simulink model "model_sim_fuzzy"  (R2023b)
settings: Solver=FixedStepAuto  StartTime=0.0  StopTime=tsim  FixedStep=T  RelTol=1e-3
values from neighbouring files (symbols this model uses):
  GIE = Ki(1) * GE(1)    [gains.m]
  GU = Kp(1) / GE(1)    [gains.m]
undefined symbols (not defined in the file or in its folder): GCE, GE, T
libraries: fuzblock x2
settings Model: Creator=usuario  LastModifiedBy=usuario
settings DataIOCC: ReturnWorkspaceOutputs=off  TimeSaveName=t

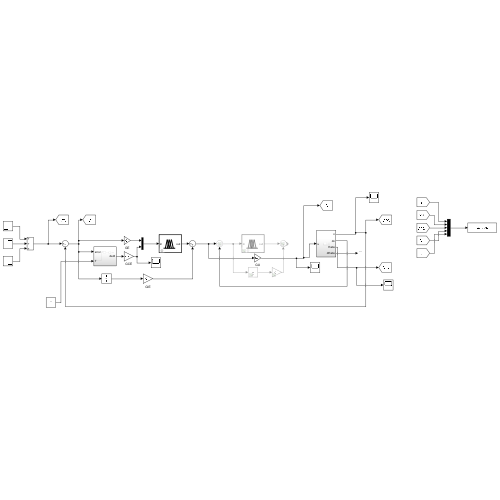
[thumbnail: Simulink's stored preview of the top-level diagram]
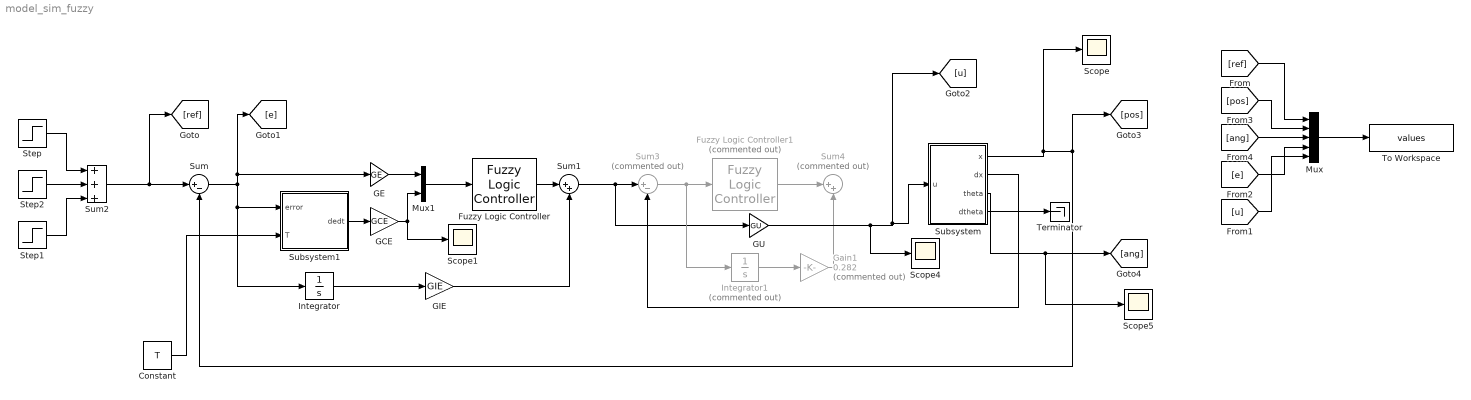
== system model_sim_fuzzy ==
  Constant : Constant  Value=T
  Fuzzy Logic Controller : fuzblock/Fuzzy Logic  Controller  FIS='PID.fis'  OutputSampleNumber=101  DataType=double  FuzzifiedInputs=off  RuleFiringStrengths=off  RuleOutputs=off  AggregatedOutputs=off  SimulateUsing=Interpreted execution  OutOfRangeInputValueMessage=warning  NoRuleFiredMessage=warning  EmptyOutputFuzzySetMessage=warning
  Fuzzy Logic Controller1 : fuzblock/Fuzzy Logic  Controller  Commented=on  FIS='PI.fis'  OutputSampleNumber=101  DataType=double  FuzzifiedInputs=off  RuleFiringStrengths=off  RuleOutputs=off  AggregatedOutputs=off  SimulateUsing=Interpreted execution  OutOfRangeInputValueMessage=warning  NoRuleFiredMessage=warning  EmptyOutputFuzzySetMessage=warning
  GCE : Gain  Gain=GCE
  GE : Gain  Gain=GE
  GIE : Gain  Gain=GIE
  GU : Gain  Gain=GU
  Gain1 : Gain  Commented=on  Gain=0.282
  Integrator : Integrator
  Integrator1 : Integrator  Commented=on
  Mux : Mux  Inputs=5
  Mux1 : Mux  Inputs=2
  Scope{,1,4..5} (4 alike) : Scope
  Step : Step  Time=0  After=0.6  SampleTime=0
  Step1 : Step  Time=30  After=-0.7  SampleTime=0
  Step2 : Step  Time=15  After=0.4  SampleTime=0
  Subsystem : Subsystem
  Subsystem1 : Subsystem
  Sum : Sum  Inputs=|+-
  Sum1 : Sum  Inputs=|++
  Sum2 : Sum  Inputs=+++
  Sum3 : Sum  Commented=on  Inputs=|+-
  Sum4 : Sum  Commented=on  Inputs=|++
  Terminator : Terminator
  To Workspace : ToWorkspace  VariableName=values  SaveFormat=Structure  SampleTime=-1
  wires:
  Mux/1 -> To Workspace/1
  Subsystem/1(x) -> Scope/1, Sum/2, [pos]
  Subsystem/3(theta) -> Scope5/1, [ang]
  Sum2/1 -> [ref], Sum/1
  Subsystem/4(dtheta) -> Terminator/1
  [ref] -> Mux/1
  [pos] -> Mux/2
  [ang] -> Mux/3
  [e] -> Mux/4
  [u] -> Mux/5
  Constant/1 -> Subsystem1/2(T)
  Sum/1 -> [e], GE/1, Integrator/1, Subsystem1/1(error)
  Step/1 -> Sum2/1
  Step1/1 -> Sum2/3
  Step2/1 -> Sum2/2
  Subsystem/2(dx) -> Sum3/2
  Mux1/1 -> Fuzzy Logic Controller/1
  Integrator/1 -> GIE/1
  GIE/1 -> Sum1/2
  Fuzzy Logic Controller/1 -> Sum1/1
  Sum1/1 -> GU/1, Sum3/1
  Sum3/1 -> Integrator1/1, Fuzzy Logic Controller1/1
  Fuzzy Logic Controller1/1 -> Sum4/1
  Integrator1/1 -> Gain1/1
  Gain1/1 -> Sum4/2
  GE/1 -> Mux1/1
  Subsystem1/1(dedt) -> GCE/1
  GCE/1 -> Mux1/2, Scope1/1
  GU/1 -> Scope4/1, [u], Subsystem/1(u)

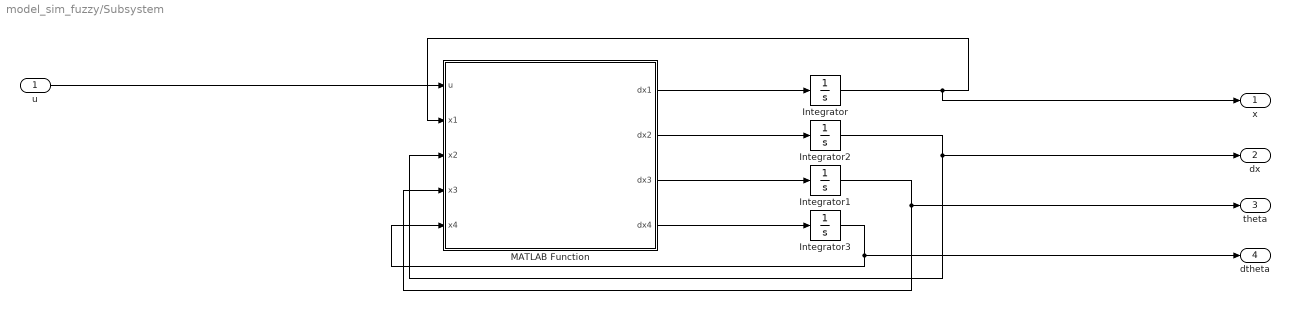
== system model_sim_fuzzy/Subsystem ==
  u : Inport
  Integrator : Integrator  InitialCondition=0.002
  Integrator1 : Integrator  InitialCondition=0.001
  Integrator2 : Integrator
  Integrator3 : Integrator
  MATLAB Function : MATLAB Function  TreatAsAtomicUnit=on
  x : Outport
  dx : Outport  Port=2
  theta : Outport  Port=3
  dtheta : Outport  Port=4
  wires:
  MATLAB Function/2(dx2) -> Integrator2/1
  Integrator/1 -> x/1, MATLAB Function/2(x1)
  Integrator2/1 -> MATLAB Function/3(x2), dx/1
  MATLAB Function/4(dx4) -> Integrator3/1
  MATLAB Function/1(dx1) -> Integrator/1
  MATLAB Function/3(dx3) -> Integrator1/1
  Integrator3/1 -> MATLAB Function/5(x4), dtheta/1
  Integrator1/1 -> theta/1, MATLAB Function/4(x3)
  u/1 -> MATLAB Function/1(u)

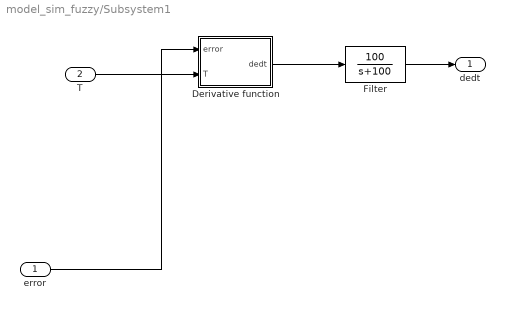
== system model_sim_fuzzy/Subsystem1 ==
  error : Inport
  T : Inport  Port=2
  Derivative function : MATLAB Function  TreatAsAtomicUnit=on  SystemSampleTime=T
  Filter : TransferFcn  Numerator=100  Denominator=[1 100]
  dedt : Outport
  wires:
  error/1 -> Derivative function/1(error)
  Derivative function/1(dedt) -> Filter/1
  T/1 -> Derivative function/2(T)
  Filter/1 -> dedt/1

== matlab function model_sim_fuzzy/Subsystem1/Derivative function ==
  data: error input; dedt output; T input
function dedt = fcn(error, T)
    persistent p_error;
    if isempty(p_error)
        p_error = error;
    end
    dedt = (error - p_error)/T;
    p_error = error;
end

== matlab function model_sim_fuzzy/Subsystem/MATLAB Function ==
  data: u input; dx1 output; x1 input; x2 input; x3 input; x4 input; dx2 output; dx3 output; dx4 output
function [dx1,dx2,dx3,dx4] = plant_model(u,x1,x2,x3,x4)
M = 10;g=9.8;m=0.8;l=0.5;mu=0.05;
q = [x1;x2;x3;x4];
a11 = -mu/(M+m*sin(x3)^2); a12 = m*g*cos(x3)*sin(x3)/((M+m*sin(x3)^2)*x3);
a13 = m*l*x4*sin(x3)/(M+m*sin(x3)^2); a21 = mu*cos(x3)/(l*(M+m*sin(x3)^2));
a22 = -(M+m)*g*sin(x3)/(l*x3*(M+m*sin(x3)^2)); a23=-m*x4*sin(x3)*cos(x3)/(M+m*sin(x3)^2);
b1 = 1/(M+m*sin(x3)^2); b2 = -cos(x3)/(l*(M+m*sin(x3)^2));
A = [0 1 0 0;0 a11 a12 a13;0 0 0 1;0 a21 a22 a23];
B = [0;b1;0;b2];

dq = A*q + B*u;
dx1 = dq(1);
dx2 = dq(2);
dx3 = dq(3);
dx4 = dq(4);
